simulink model "moyenneur"  (R2020a)
settings: Solver=VariableStepAuto  StartTime=0.0  StopTime=14  RelTol=1e-3
libraries: dspspect3 x1
settings Model: Creator=XPS 15  LastModifiedBy=XPS 15

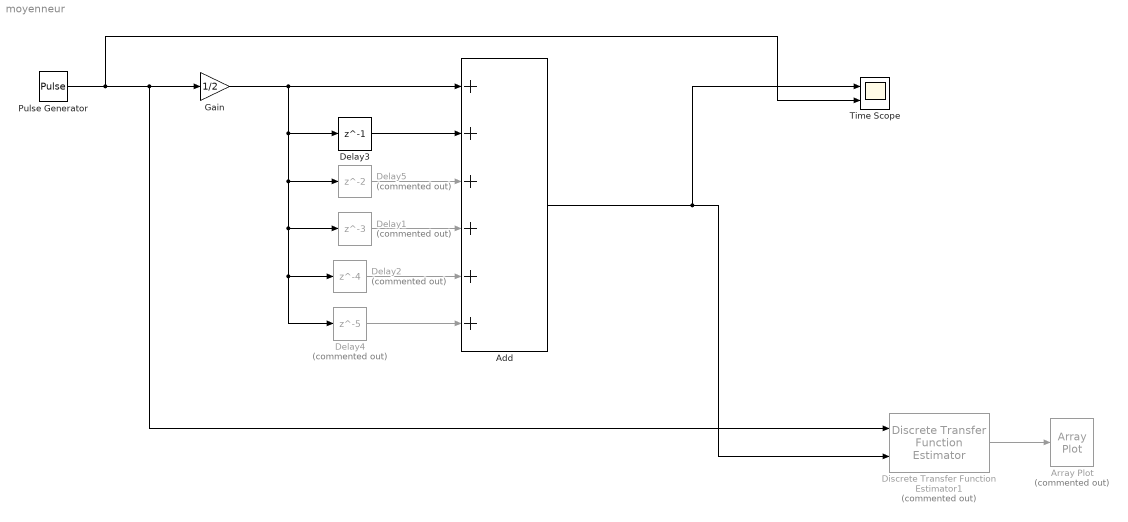
== system moyenneur ==
  Add : Sum  Inputs=++++++
  Array Plot : ArrayPlot  Commented=on
  Delay1 : Delay  Commented=on  DelayLength=3  InitialCondition=0  InputProcessing=Columns as channels (frame based)
  Delay2 : Delay  Commented=on  DelayLength=4  InitialCondition=0  InputProcessing=Columns as channels (frame based)
  Delay3 : Delay  DelayLength=1  InitialCondition=0
  Delay4 : Delay  Commented=on  DelayLength=5  InitialCondition=0  InputProcessing=Columns as channels (frame based)
  Delay5 : Delay  Commented=on  InitialCondition=0  InputProcessing=Columns as channels (frame based)
  Discrete Transfer Function Estimator1 : dspspect3/Discrete Transfer Function Estimator  Commented=on  WindowMode=Specify on dialog  WindowLength=1024  Overlap=50  AveragingMethod=Running  ForgettingFactorPort=off  ForgettingFactor=0.9  SpectralAverages=100  FFTLengthSource=Auto  FFTLength=128  Window=Hann  SidelobeAttenuation=60  FrequencyRange=One-sided  OutputCoherence=off  SimulateUsing=Code generation
      settings: SourceProductBaseCode=DS
  Gain : Gain  Gain=1/2
  Pulse Generator : DiscretePulseGenerator  Period=24*6  SampleTime=1/24
  Time Scope : Scope  NumInputPorts=2
  wires:
  Delay3/1 -> Add/2
  Discrete Transfer Function Estimator1/1 -> Array Plot/1
  Add/1 -> Time Scope/1, Discrete Transfer Function Estimator1/2
  Gain/1 -> Delay5/1, Delay4/1, Delay2/1, Delay1/1, Delay3/1, Add/1
  Delay2/1 -> Add/5
  Pulse Generator/1 -> Time Scope/2, Discrete Transfer Function Estimator1/1, Gain/1
  Delay1/1 -> Add/4
  Delay5/1 -> Add/3
  Delay4/1 -> Add/6
